simulink model "Simulador"  (R2015a)
settings: Solver=ode45  StartTime=0.0  StopTime=Inf  MaxStep=1  RelTol=1e-3
StopFcn:
  | close all
  | post_simulacion
model workspace (MAT data in the model file):
  m = 3.797
  b = 2.1
  c = 0.3571
  Salar = 0.75
  AR = 5.88
  cg = [0.44 0 0]
  Ix = 1.229
  Iy = 0.1702
  Iz = 0.8808
  Ixz = 0.9343
  e = 0.9935
  alpha0 = 0.267
  coefprop = [0.016415 -0.0142726]
  C_L0 = 0.0254
  C_Lalpha = 4.0191
  C_Lq = 3.8954
  C_Ldelta_e = 0.5872
  C_D0 = 0.0102
  C_Dbeta1 = -2.0864e-07
  C_Dbeta2 = 0.0671
  C_Dq = 0
  C_Ddelta_e = 0.8461
  C_Y0 = 3.2049e-18
  C_Ybeta = -0.1949
  C_Yp = -0.1172
  C_Yr = 0.0959
  C_Ydelta_a = -0.0696
  C_l0 = 1.1518e-18
  C_lbeta = -0.0765
  C_lp = -0.4018
  C_lr = 0.025
  C_ldelta_a = 0.2987
  C_m0 = 0.018
  C_malpha = -0.2524
  C_mq = -1.3047
  C_mdelta_e = -0.4857
  C_n0 = -2.2667e-07
  C_nbeta = 0.0403
  C_np = -0.0247
  C_nr = -0.1252
  C_ndelta_a = 0.0076
  gamma = 0.20958671
  gamma1 = 8.64638926772
  gamma2 = 7.15127867602
  gamma3 = 4.20255654569
  gamma4 = 4.4578208227
  gamma5 = -2.04582843713
  gamma6 = 5.48942420682
  gamma7 = 10.3736620037
  gamma8 = 5.86392142899
  C_p0 = -1.01045424588e-06
  C_pbeta = -0.14184539659
  C_pp = -1.79869539438
  C_pr = -0.45305525336
  C_pdelta_a = 1.28918307845
  C_r0 = -1.3291750703e-06
  C_rbeta = -0.104707259349
  C_rp = -1.93599126586
  C_rr = -0.622717442342
  C_rdelta_a = 1.3761168826
  C_mp = -0.2168
values from neighbouring files (symbols this model uses):
  r = [r_n;r_e;r_d]    [segmento.m]
  waypoints = reshape(waypoints_mat.',[],1)    [plan_de_vuelo.m]
undefined symbols (not defined in the file or in its folder): F, Light, magnitude, MIL, plan_de_vuelo
libraries: simulink_extras x20, aerolibconvert2 x18, aerolibfltsims x2, simulink x2, vrlib x1, instrumentlib x1, aerolibatmos2 x1, aerolibtransform2 x1, aerolibwind2 x1, aerolibgravity2 x1
(part 1 of 3)
settings Model: TunableVars=Velocidad_aerodinamica_AP,Rumbo_AP,Altitud_AP,PalancaTeclado,FMS,GNSS,Viento  TunableVarsStorageClass=Auto,Auto,Auto,Auto,Auto,Auto,Auto  TunableVarsTypeQualifier=,,,,,,  Creator=Cecilia Ruiz Romero  LastModifiedBy=Cecilia Ruiz Romero
settings DataIOCC: TimeSaveName=tiempos

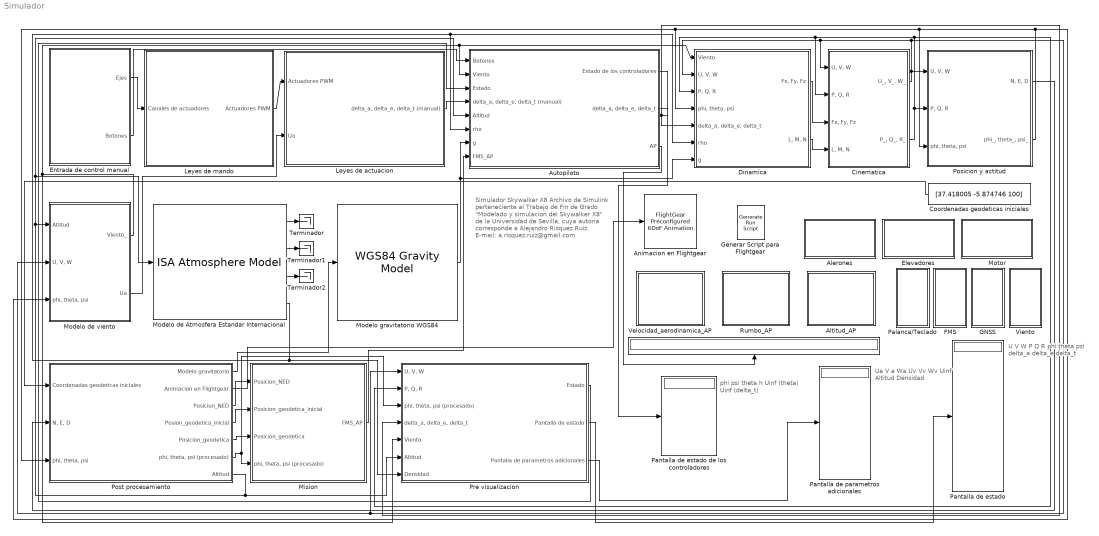
== system Simulador ==
  note: U
      | V
      | W
      | P
      | Q
      | R
      | phi
      | theta
      | psi
      | delta_a
      | delta_e
      | delta_t
  note: Ua
      | V a
      | Wa
      | Uv
      | Vv
      | Wv
      | Uinf
      | Altitud
      | Densidad
  note: phi
      | psi
      | theta
      | h
      | Uinf (theta)
      | Uinf (delta_t)
  note: Simulador Skywalker X8
      |
      | Archivo de Simulink perteneciente al Trabajo de Fin de Grado "Modelado y simulacion del Skywalker X8" de la Universidad de Sevilla, cuya autoria corresponde a Alejandro Risquez Ruiz.
      |
      | E-mail: a.risquez.ruiz@gmail.com
  " " : Display
  Alerones : Subsystem  DialogController=hmiCreateDDGDialog  IsWebBlock=on  mask(MathWorksWebBlock){webBlockId=14687f7d-6eed-453e-adcd-d1944eb0612c, webBlockType=semicirculargauge, ShowInLibBrowser=on, ShowInitialText=on, HMISrcModelName=Simulador}
      mask prompts: webBlockId "WebBlock Id"; webBlockType "WebBlock Type"; HMISrcModelName "Source Model"
      mask Help: helpview([docroot '/mapfiles/simulink.map'], 'hmi_half_gauge')
      mask Display:
      | if strcmp(get_param(bdroot(gcb),'BlockDiagramType'), 'library')
      |     image([(matlabroot) '/toolbox/simulink/hmi/icons/SemicircularGauge.png']);
      | end
  Altitud_AP : Subsystem  DialogController=hmiCreateDDGDialog  IsWebBlock=on  mask(MathWorksWebBlock){webBlockId=223b671f-8fe1-4181-b377-fa138c1070ca, webBlockType=continuousknob, ShowInLibBrowser=on, ShowInitialText=on, HMISrcModelName=Simulador}
      mask prompts: webBlockId "WebBlock Id"; webBlockType "WebBlock Type"; HMISrcModelName "Source Model"
      mask Help: helpview([docroot '/mapfiles/simulink.map'], 'hmi_knob')
      mask Display:
      | if strcmp(get_param(bdroot(gcb),'BlockDiagramType'), 'library')
      |     image([(matlabroot) '/toolbox/simulink/hmi/icons/ContinuousKnob.png']);
      | end
  Animacion en Flightgear : aerolibfltsims/FlightGear Preconfigured 6DoF Animation  xFlightGearVersion=v3.0  DestinationIpAddress=192.168.1.33  DestinationPort=5502  SampleTime=1/30
  Autopiloto : Subsystem
  Cinematica : Subsystem
  Coordenadas geodeticas iniciales : Constant  Value=[37.418005 -5.874746 100]
  Dinamica : Subsystem
  Elevadores : Subsystem  DialogController=hmiCreateDDGDialog  IsWebBlock=on  mask(MathWorksWebBlock){webBlockId=d989d251-72c9-40e1-9d1b-cd89d142c18d, webBlockType=semicirculargauge, ShowInLibBrowser=on, ShowInitialText=on, HMISrcModelName=Simulador}
      mask prompts: webBlockId "WebBlock Id"; webBlockType "WebBlock Type"; HMISrcModelName "Source Model"
      mask Help: helpview([docroot '/mapfiles/simulink.map'], 'hmi_half_gauge')
      mask Display:
      | if strcmp(get_param(bdroot(gcb),'BlockDiagramType'), 'library')
      |     image([(matlabroot) '/toolbox/simulink/hmi/icons/SemicircularGauge.png']);
      | end
  Entrada de control manual : Subsystem
  FMS : Subsystem  DialogController=hmiCreateDDGDialog  IsWebBlock=on  mask(MathWorksWebBlock){webBlockId=f65861c9-849a-4d55-a765-84128246603e, webBlockType=toggleswitch, ShowInLibBrowser=on, ShowInitialText=on, HMISrcModelName=Simulador}
      mask prompts: webBlockId "WebBlock Id"; webBlockType "WebBlock Type"; HMISrcModelName "Source Model"
      mask Help: helpview([docroot '/mapfiles/simulink.map'], 'hmi_toggle_switch')
      mask Display:
      | if strcmp(get_param(bdroot(gcb),'BlockDiagramType'), 'library')
      |     image([(matlabroot) '/toolbox/simulink/hmi/icons/ToggleSwitch.png']);
      | end
  GNSS : Subsystem  DialogController=hmiCreateDDGDialog  IsWebBlock=on  mask(MathWorksWebBlock){webBlockId=2f82c36a-ef1f-4a61-96ee-8f2028b7861b, webBlockType=toggleswitch, ShowInLibBrowser=on, ShowInitialText=on, HMISrcModelName=Simulador}
      mask prompts: webBlockId "WebBlock Id"; webBlockType "WebBlock Type"; HMISrcModelName "Source Model"
      mask Help: helpview([docroot '/mapfiles/simulink.map'], 'hmi_toggle_switch')
      mask Display:
      | if strcmp(get_param(bdroot(gcb),'BlockDiagramType'), 'library')
      |     image([(matlabroot) '/toolbox/simulink/hmi/icons/ToggleSwitch.png']);
      | end
  Generar Script para Flightgear : aerolibfltsims/Generate Run Script  OutputFileName=Flightgear_simulador.bat  FlightGearBaseDirectory=C:\Program Files\FlightGear  GeometryModelName=Malolo1  DestinationPort=5502  OriginAddress=192.168.1.34  OriginPort=5505  LocalAddress=192.168.1.35  AirportId=LEZL  RunwayId=27  InitialAltitude=328  InitialHeading=270  OffsetDistance=0  OffsetAzimuth=0  GenerateFile=off  Architecture=Win64  dataFlow=Receive
  Leyes de actuacion : Subsystem
  Leyes de mando : Subsystem
  Mision : Subsystem
  Modelo de Atmosfera Estandar Internacional : aerolibatmos2/ISA Atmosphere Model  custom=off  g=9.80665  gamma=1.4  R=287.0531  L=0.0065  h_trop=11000  h_strat=20000  rho0=1.225  P0=101325  T0=288.15  h0=0
  Modelo de viento : Subsystem
  Modelo gravitatorio WGS84 : aerolibgravity2/WGS84 Gravity Model   model=WGS84 Taylor Series  units=Metric (MKS)  no_atmos=on  precessing=on  jd_loc=off  month=October  day=10  year=2004  no_centrifugal=on  action=Warning
  Motor : Subsystem  DialogController=hmiCreateDDGDialog  IsWebBlock=on  mask(MathWorksWebBlock){webBlockId=dc943369-9c23-4275-9e07-e512671338e7, webBlockType=semicirculargauge, ShowInLibBrowser=on, ShowInitialText=on, HMISrcModelName=Simulador}
      mask prompts: webBlockId "WebBlock Id"; webBlockType "WebBlock Type"; HMISrcModelName "Source Model"
      mask Help: helpview([docroot '/mapfiles/simulink.map'], 'hmi_half_gauge')
      mask Display:
      | if strcmp(get_param(bdroot(gcb),'BlockDiagramType'), 'library')
      |     image([(matlabroot) '/toolbox/simulink/hmi/icons/SemicircularGauge.png']);
      | end
  Palanca/Teclado : Subsystem  DialogController=hmiCreateDDGDialog  IsWebBlock=on  mask(MathWorksWebBlock){webBlockId=b63e11f2-ce41-4b45-96ee-a8e10d270359, webBlockType=toggleswitch, ShowInLibBrowser=on, ShowInitialText=on, HMISrcModelName=Simulador}
      mask prompts: webBlockId "WebBlock Id"; webBlockType "WebBlock Type"; HMISrcModelName "Source Model"
      mask Help: helpview([docroot '/mapfiles/simulink.map'], 'hmi_toggle_switch')
      mask Display:
      | if strcmp(get_param(bdroot(gcb),'BlockDiagramType'), 'library')
      |     image([(matlabroot) '/toolbox/simulink/hmi/icons/ToggleSwitch.png']);
      | end
  Pantalla de estado : Display
  Pantalla de estado de los controladores : Display
  Pantalla de parametros adicionales : Display
  Posicion y actitud : Subsystem
  Post procesamiento : Subsystem
  Pre visualizacion : Subsystem
  Rumbo_AP : Subsystem  DialogController=hmiCreateDDGDialog  IsWebBlock=on  mask(MathWorksWebBlock){webBlockId=9d5373b8-7b64-41e6-bd7e-2392d6322634, webBlockType=continuousknob, ShowInLibBrowser=on, ShowInitialText=on, HMISrcModelName=Simulador}
      mask prompts: webBlockId "WebBlock Id"; webBlockType "WebBlock Type"; HMISrcModelName "Source Model"
      mask Help: helpview([docroot '/mapfiles/simulink.map'], 'hmi_knob')
      mask Display:
      | if strcmp(get_param(bdroot(gcb),'BlockDiagramType'), 'library')
      |     image([(matlabroot) '/toolbox/simulink/hmi/icons/ContinuousKnob.png']);
      | end
  Terminador : Terminator
  Terminador1 : Terminator
  Terminador2 : Terminator
  Velocidad_aerodinamica_AP : Subsystem  DialogController=hmiCreateDDGDialog  IsWebBlock=on  mask(MathWorksWebBlock){webBlockId=5a147658-4b96-4464-a5e7-82583d5f87ac, webBlockType=continuousknob, ShowInLibBrowser=on, ShowInitialText=on, HMISrcModelName=Simulador}
      mask prompts: webBlockId "WebBlock Id"; webBlockType "WebBlock Type"; HMISrcModelName "Source Model"
      mask Help: helpview([docroot '/mapfiles/simulink.map'], 'hmi_knob')
      mask Display:
      | if strcmp(get_param(bdroot(gcb),'BlockDiagramType'), 'library')
      |     image([(matlabroot) '/toolbox/simulink/hmi/icons/ContinuousKnob.png']);
      | end
  Viento : Subsystem  DialogController=hmiCreateDDGDialog  IsWebBlock=on  mask(MathWorksWebBlock){webBlockId=de649073-e8b6-4552-a188-ccf5b7e05afd, webBlockType=toggleswitch, ShowInLibBrowser=on, ShowInitialText=on, HMISrcModelName=Simulador}
      mask prompts: webBlockId "WebBlock Id"; webBlockType "WebBlock Type"; HMISrcModelName "Source Model"
      mask Help: helpview([docroot '/mapfiles/simulink.map'], 'hmi_toggle_switch')
      mask Display:
      | if strcmp(get_param(bdroot(gcb),'BlockDiagramType'), 'library')
      |     image([(matlabroot) '/toolbox/simulink/hmi/icons/ToggleSwitch.png']);
      | end
  wires:
  Entrada de control manual/1(Ejes) -> Leyes de mando/1(Canales de actuadores)
  Entrada de control manual/2(Botones) -> Autopiloto/1(Botones)
  Leyes de mando/1(Actuadores PWM) -> Leyes de actuacion/1(Actuadores PWM)
  Modelo de Atmosfera Estandar Internacional/1 -> Terminador/1
  Modelo de Atmosfera Estandar Internacional/2 -> Terminador1/1
  Modelo de Atmosfera Estandar Internacional/3 -> Terminador2/1
  Pre visualizacion/1(Estado) -> Autopiloto/3(Estado)
  Leyes de actuacion/1("delta_a, delta_e, delta_t (manual)") -> Autopiloto/4("delta_a, delta_e, delta_t (manual)")
  Post procesamiento/7(Altitud) -> Modelo de viento/1(Altitud), Modelo de Atmosfera Estandar Internacional/1, Autopiloto/5(Altitud), Pre visualizacion/6(Altitud)
  Mision/1(FMS_AP) -> Autopiloto/8(FMS_AP)
  Autopiloto/2("delta_a, delta_e, delta_t") -> Pre visualizacion/4("delta_a, delta_e, delta_t"), Dinamica/5("delta_a, delta_e, delta_t")
  Cinematica/1("U_, V_, W_") -> Posicion y actitud/1("U, V, W"), Modelo de viento/2("U, V, W"), Pre visualizacion/1("U, V, W"), Cinematica/1("U, V, W"), Dinamica/2("U, V, W")
  Modelo de viento/1(Viento_) -> Pre visualizacion/5(Viento), Dinamica/1(Viento), Autopiloto/2(Viento)
  Modelo de Atmosfera Estandar Internacional/4 -> Pre visualizacion/7(Densidad), Dinamica/6(rho), Autopiloto/6(rho)
  Autopiloto/1(Estado de los controladores) -> Pantalla de estado de los controladores/1
  Cinematica/2("P_, Q_, R_") -> Posicion y actitud/2("P, Q, R"), Pre visualizacion/2("P, Q, R"), Cinematica/2("P, Q, R"), Dinamica/3("P, Q, R")
  Posicion y actitud/2("phi_, theta_, psi_") -> Posicion y actitud/3("phi, theta, psi"), Dinamica/4("phi, theta, psi"), Post procesamiento/3("phi, theta, psi"), Modelo de viento/3("phi, theta, psi")
  Autopiloto/3(AP) -> " "/1
  Dinamica/1("Fx, Fy, Fz") -> Cinematica/3("Fx, Fy, Fz")
  Dinamica/2("L, M, N") -> Cinematica/4("L, M, N")
  Posicion y actitud/1("N, E, D") -> Post procesamiento/2("N, E, D")
  Coordenadas geodeticas iniciales/1 -> Post procesamiento/1(Coordenadas geodeticas iniciales)
  Post procesamiento/2(Animacion en Flightgear) -> Animacion en Flightgear/1
  Post procesamiento/3(Posicion_NED) -> Mision/1(Posicion_NED)
  Post procesamiento/4(Posion_geodetica_inicial) -> Mision/2(Posicion_geodetica_inicial)
  Post procesamiento/5(Posicion_geodetica) -> Mision/3(Posicion_geodetica)
  Post procesamiento/6("phi, theta, psi (procesado)") -> Mision/4("phi, theta, psi (procesado)"), Pre visualizacion/3("phi, theta, psi (procesado)")
  Pre visualizacion/2(Pantalla de estado) -> Pantalla de estado/1
  Pre visualizacion/3(Pantalla de parametros adicionales) -> Pantalla de parametros adicionales/1
  Modelo de viento/2(Ua) -> Leyes de actuacion/2(Ua)
  Modelo gravitatorio WGS84/1 -> Dinamica/7(g), Autopiloto/7(g)
  Post procesamiento/1(Modelo gravitatorio) -> Modelo gravitatorio WGS84/1

== system Simulador/Alerones ==

== system Simulador/Altitud_AP ==

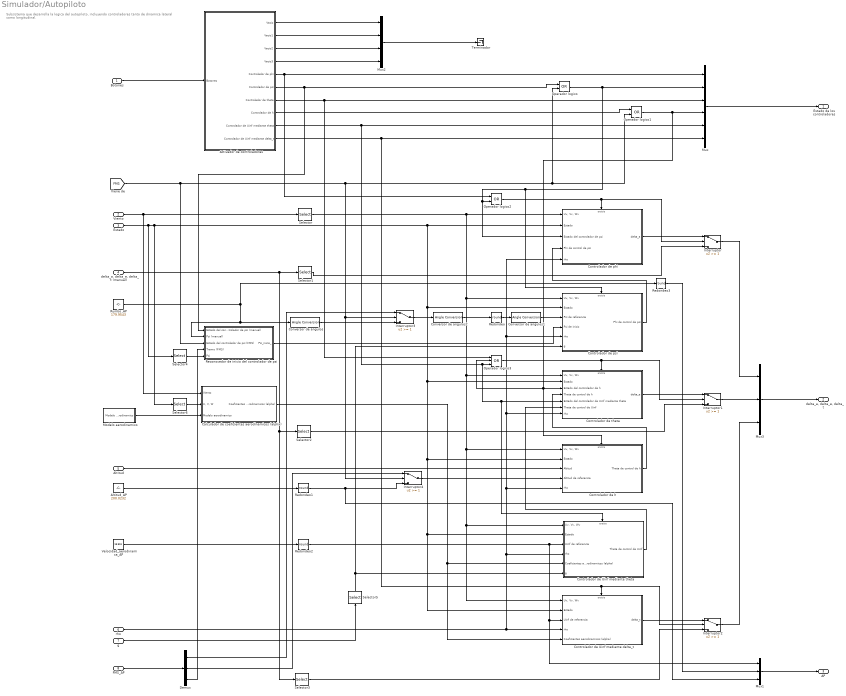
== system Simulador/Autopiloto ==
  note: Subsistema que desarrolla la logica del
      | autopiloto, incluyendo controladores tanto
      | de dinamica lateral como longitudinal.
  Botones : Inport
  Viento : Inport  Port=2
  Estado : Inport  Port=3
  "delta_a, delta_e, delta_t (manual)" : Inport  Port=4
  Altitud : Inport  Port=5
  rho : Inport  Port=6
  g : Inport  Port=7
  FMS_AP : Inport  Port=8
  Activador de controladores : Subsystem
  Altitud_AP : Constant  Value=200.0232
  Calculador de coeficientes aerodinamicos (alpha) : Subsystem
  Controlador de Uinf mediante delta_t : Subsystem
  Controlador de Uinf mediante theta : Subsystem
  Controlador de h : Subsystem
  Controlador de phi : Subsystem
  Controlador de psi : Subsystem
  Controlador de theta : Subsystem
  Conversor de angulos : aerolibconvert2/Angle Conversion  IU=deg  OU=rad
  Conversor de angulos1 : aerolibconvert2/Angle Conversion  IU=deg  OU=rad
  Conversor de angulos2 : aerolibconvert2/Angle Conversion  IU=rad  OU=deg
  Demux : Demux  Outputs=3
  Interruptor{,1..4} (5 alike) : Switch  Threshold=1
  Modelo aerodinamico : Subsystem
  Mux : Mux  Inputs=6
  Mux1 : Mux  Inputs=3
  Mux2 : Mux
  Mux3 : Mux  Inputs=3
  Operador logico : Logic  Operator=OR  AllPortsSameDT=off  OutDataTypeStr=boolean
  Operador logico1 : Logic  Operator=OR  AllPortsSameDT=off  OutDataTypeStr=boolean
  Operador logico2 : Logic  Operator=OR  AllPortsSameDT=off  OutDataTypeStr=boolean
  Operador logico3 : Logic  Operator=OR  Inputs=3  AllPortsSameDT=off  OutDataTypeStr=boolean
  Reconocedor de inicio del controlador de psi : Subsystem
  Redondeo{,1..3} (4 alike) : Rounding  Operator=round
  Rumbo_AP : Constant  Value=179.9543
  Selector : Selector  InputPortWidth=6  Indices=[1 2 3]
  Selector1 : Selector  InputPortWidth=3
  Selector2 : Selector  InputPortWidth=3  Indices=2
  Selector3 : Selector  InputPortWidth=3  Indices=3
  Selector4 : Selector  InputPortWidth=12  Indices=9
  Selector5 : Selector  InputPortWidth=3  Indices=3
  Selector6 : Selector  InputPortWidth=12  Indices=[1 2 3]
  Terminador : Terminator
  Velocidad_aerodinamica_AP : Constant  Value=19.919
  Estado de los controladores : Outport
  "delta_a, delta_e, delta_t" : Outport  Port=2
  AP : Outport  Port=3
  wires:
  Botones/1 -> Activador de controladores/1(Botones)
  Mux1/1 -> AP/1
  Altitud_AP/1 -> Redondeo1/1
  [FMS] -> Operador logico1/2, Operador logico/2, Interruptor4/2, Interruptor3/2, Reconocedor de inicio del controlador de psi/3(Estado del controlador de psi (FMS))
  Activador de controladores/9(Controlador de Uinf mediante theta) -> Mux/5, Controlador de theta/5(Estado del controlador de Uinf mediante theta), Controlador de Uinf mediante theta/Enable, Operador logico3/3
  Activador de controladores/8(Controlador de h) -> Operador logico1/1
  Activador de controladores/7(Controlador de theta) -> Mux/3, Operador logico3/1
  Activador de controladores/5(Controlador de phi) -> Mux/1, Operador logico2/1
  Activador de controladores/6(Controlador de psi) -> Operador logico/1, Reconocedor de inicio del controlador de psi/1(Estado del controlador de psi (manual))
  Activador de controladores/1(Vacio) -> Mux2/1
  Activador de controladores/2(Vacio1) -> Mux2/2
  Activador de controladores/3(Vacio2) -> Mux2/3
  Activador de controladores/4(Vacio3) -> Mux2/4
  Mux2/1 -> Terminador/1
  Mux/1 -> Estado de los controladores/1
  Viento/1 -> Calculador de coeficientes aerodinamicos (alpha)/1(Viento), Selector/1
  Estado/1 -> Selector6/1, Controlador de Uinf mediante delta_t/2("Estado "), Controlador de Uinf mediante theta/2("Estado "), Controlador de h/2("Estado "), Controlador de theta/2("Estado "), Controlador de psi/2("Estado "), Controlador de phi/2("Estado "), Selector4/1
  Selector/1 -> Controlador de Uinf mediante delta_t/1("Uv, Vv, Wv"), Controlador de Uinf mediante theta/1("Uv, Vv, Wv"), Controlador de h/1("Uv, Vv, Wv"), Controlador de theta/1("Uv, Vv, Wv"), Controlador de psi/1("Uv, Vv, Wv"), Controlador de phi/1("Uv, Vv, Wv")
  Operador logico2/1 -> Interruptor/2, Controlador de phi/Enable
  Controlador de phi/1(delta_a) -> Interruptor/1
  "delta_a, delta_e, delta_t (manual)"/1 -> Selector1/1, Selector2/1, Selector3/1
  Selector1/1 -> Interruptor/3
  Controlador de psi/1(Phi de control de psi) -> Controlador de phi/4(Phi de control de psi)
  Operador logico3/1 -> Interruptor1/2, Controlador de theta/Enable
  Controlador de theta/1(delta_e) -> Interruptor1/1
  Selector2/1 -> Interruptor1/3
  rho/1 -> Controlador de Uinf mediante delta_t/4(rho), Controlador de h/5(rho), Controlador de theta/7(rho), Controlador de psi/5(rho), Controlador de phi/5(rho), Controlador de Uinf mediante theta/4(rho)
  Controlador de h/1(Theta de control de h) -> Controlador de theta/4(Theta de control de h)
  Redondeo2/1 -> Mux1/1, Controlador de Uinf mediante delta_t/3(Uinf de referencia), Controlador de Uinf mediante theta/3(Uinf de referencia)
  Velocidad_aerodinamica_AP/1 -> Redondeo2/1
  Activador de controladores/10(Controlador de Uinf mediante delta_t) -> Mux/6, Controlador de Uinf mediante delta_t/Enable, Interruptor2/2
  Controlador de Uinf mediante delta_t/1(delta_t) -> Interruptor2/1
  Selector3/1 -> Interruptor2/3
  Controlador de Uinf mediante theta/1(Theta de control de Uinf) -> Controlador de theta/6(Theta de control de Uinf)
  Altitud/1 -> Controlador de h/3(Altitud)
  Interruptor4/1 -> Controlador de h/4(Altitud de referencia)
  Mux3/1 -> "delta_a, delta_e, delta_t"/1
  Interruptor2/1 -> Mux3/3
  Interruptor1/1 -> Mux3/2
  Interruptor/1 -> Mux3/1
  Redondeo1/1 -> Mux1/3, Interruptor4/3
  Redondeo3/1 -> Mux1/2
  FMS_AP/1 -> Demux/1
  Rumbo_AP/1 -> Redondeo3/1, Conversor de angulos/1, Reconocedor de inicio del controlador de psi/2(Psi (manual))
  Selector4/1 -> Reconocedor de inicio del controlador de psi/5(Psi)
  Reconocedor de inicio del controlador de psi/1(Psi_inicio_) -> Controlador de psi/4(Psi de inicio)
  Operador logico/1 -> Mux/2, Operador logico2/2, Controlador de phi/3(Estado del controlador de psi), Controlador de psi/Enable
  Operador logico1/1 -> Controlador de theta/3(Estado del controlador de h), Operador logico3/2, Controlador de h/Enable, Mux/4
  Conversor de angulos1/1 -> Controlador de psi/3(Psi de referencia)
  Redondeo/1 -> Conversor de angulos1/1
  Conversor de angulos/1 -> Interruptor3/3
  Conversor de angulos2/1 -> Redondeo/1
  Interruptor3/1 -> Conversor de angulos2/1
  g/1 -> Selector5/1
  Selector5/1 -> Controlador de psi/6(g), Controlador de Uinf mediante theta/6(g)
  Modelo aerodinamico/1(Modelo aerodinamico) -> Calculador de coeficientes aerodinamicos (alpha)/3(Modelo aerodinamico)
  Selector6/1 -> Calculador de coeficientes aerodinamicos (alpha)/2("U, V, W")
  Calculador de coeficientes aerodinamicos (alpha)/1(Coeficientes aerodinamicos (alpha)) -> Controlador de Uinf mediante delta_t/5(Coeficientes aerodinamicos (alpha)), Controlador de Uinf mediante theta/5(Coeficientes aerodinamicos (alpha))
  Demux/3 -> Reconocedor de inicio del controlador de psi/4(Tramo (FMS))
  Demux/1 -> Interruptor3/1
  Demux/2 -> Interruptor4/1

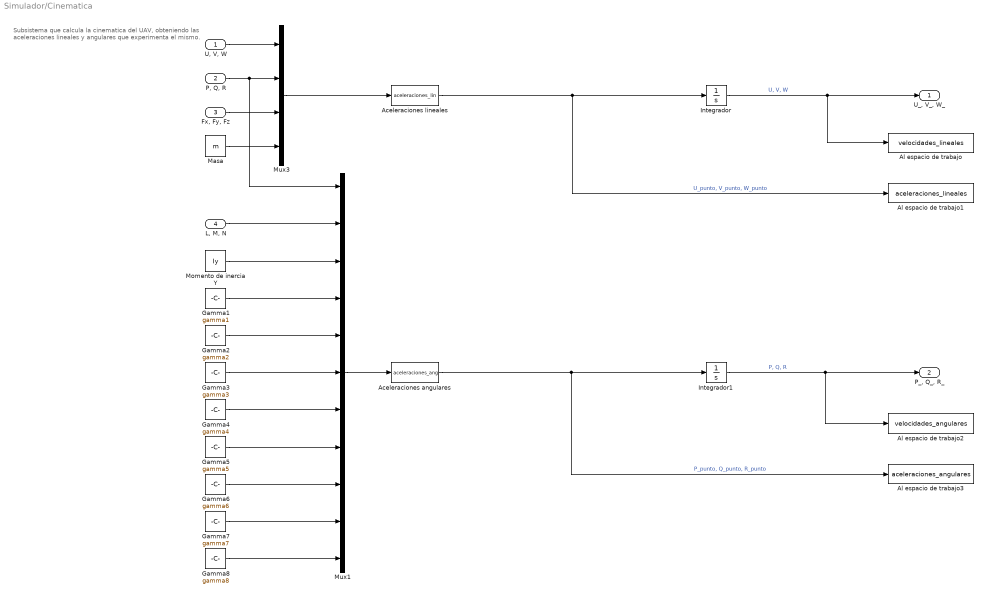
== system Simulador/Cinematica ==
  note: Subsistema que calcula la cinematica del
      | UAV, obteniendo las aceleraciones lineales
      | y angulares que experimenta el mismo.
  "U, V, W" : Inport
  "P, Q, R" : Inport  Port=2
  "Fx, Fy, Fz" : Inport  Port=3
  "L, M, N" : Inport  Port=4
  Aceleraciones angulares : MATLABFcn  MATLABFcn=aceleraciones_ang  OutputDimensions=3
  Aceleraciones lineales : MATLABFcn  MATLABFcn=aceleraciones_lin  OutputDimensions=3
  Al espacio de trabajo : ToWorkspace  VariableName=velocidades_lineales  SaveFormat=Timeseries  SampleTime=-1
  Al espacio de trabajo1 : ToWorkspace  VariableName=aceleraciones_lineales  SaveFormat=Timeseries  SampleTime=-1
  Al espacio de trabajo2 : ToWorkspace  VariableName=velocidades_angulares  SaveFormat=Timeseries  SampleTime=-1
  Al espacio de trabajo3 : ToWorkspace  VariableName=aceleraciones_angulares  SaveFormat=Timeseries  SampleTime=-1
  Gamma1 : Constant  Value=gamma1
  Gamma2 : Constant  Value=gamma2
  Gamma3 : Constant  Value=gamma3
  Gamma4 : Constant  Value=gamma4
  Gamma5 : Constant  Value=gamma5
  Gamma6 : Constant  Value=gamma6
  Gamma7 : Constant  Value=gamma7
  Gamma8 : Constant  Value=gamma8
  Integrador : Integrator  InitialCondition=[22.5000 1.20777e-04 0.678706]
  Integrador1 : Integrator  InitialCondition=[-6.87125e-22 -3.91163e-24 -2.13625e-23]
  Masa : Constant  Value=m
  Momento de inercia Y : Constant  Value=Iy
  Mux1 : Mux  Inputs=11
  Mux3 : Mux
  "U_, V_, W_" : Outport
  "P_, Q_, R_" : Outport  Port=2
  wires:
  Aceleraciones lineales/1 -> Integrador/1, Al espacio de trabajo1/1  "U_punto, V_punto, W_punto"
  Aceleraciones angulares/1 -> Integrador1/1, Al espacio de trabajo3/1  "P_punto, Q_punto, R_punto"
  "U, V, W"/1 -> Mux3/1
  "P, Q, R"/1 -> Mux3/2, Mux1/1
  "Fx, Fy, Fz"/1 -> Mux3/3
  "L, M, N"/1 -> Mux1/2
  Mux3/1 -> Aceleraciones lineales/1
  Mux1/1 -> Aceleraciones angulares/1
  Integrador/1 -> "U_, V_, W_"/1, Al espacio de trabajo/1  "U, V, W"
  Integrador1/1 -> "P_, Q_, R_"/1, Al espacio de trabajo2/1  "P, Q, R"
  Momento de inercia Y/1 -> Mux1/3
  Gamma1/1 -> Mux1/4
  Gamma2/1 -> Mux1/5
  Gamma3/1 -> Mux1/6
  Gamma4/1 -> Mux1/7
  Gamma5/1 -> Mux1/8
  Gamma6/1 -> Mux1/9
  Gamma7/1 -> Mux1/10
  Gamma8/1 -> Mux1/11
  Masa/1 -> Mux3/4

== system Simulador/Dinamica ==
  note: Subsistema que calcula la dinamica
      | del UAV, obteniendo las fuerzas y
      | momentos ejercidos sobre el mismo.
  Viento : Inport
  "U, V, W" : Inport  Port=2
  "P, Q, R" : Inport  Port=3
  "phi, theta, psi" : Inport  Port=4
  "delta_a, delta_e, delta_t" : Inport  Port=5
  rho : Inport  Port=6
  g : Inport  Port=7
  Al espacio de trabajo : ToWorkspace  VariableName=fuerzas  SaveFormat=Timeseries  SampleTime=-1
  Al espacio de trabajo1 : ToWorkspace  VariableName=momentos  SaveFormat=Timeseries  SampleTime=-1
  Calculador de coeficientes aerodinamicos : Subsystem
  Fuerzas : MATLABFcn  MATLABFcn=fuerzas  OutputDimensions=3
  Modelo aerodinamico : Subsystem
  Momentos : MATLABFcn  MATLABFcn=momentos  OutputDimensions=3
  Mux1 : Mux  Inputs=10
  Mux5 : Mux  Inputs=6
  Selector : Selector  InputPortWidth=6  Indices=[1 2 3]
  Selector1 : Selector  InputPortWidth=3  Indices=3
  Selector2 : Selector  InputPortWidth=3  Indices=3
  Selector3 : Selector  InputPortWidth=35
  Selector4 : Selector  InputPortWidth=35  Indices=4
  Selector5 : Selector  InputPortWidth=6  Indices=[4 5 6]
  Selector6 : Selector  InputPortWidth=35  Indices=2
  Selector7 : Selector  InputPortWidth=35  Indices=3
  "Fx, Fy, Fz" : Outport
  "L, M, N" : Outport  Port=2
  wires:
  Fuerzas/1 -> "Fx, Fy, Fz"/1, Al espacio de trabajo/1  "Fx, Fy, Fz"
  Momentos/1 -> "L, M, N"/1, Al espacio de trabajo1/1  "L, M, N"
  g/1 -> Selector2/1
  "delta_a, delta_e, delta_t"/1 -> Selector1/1, Calculador de coeficientes aerodinamicos/4("delta_a, delta_e, delta_t")
  Viento/1 -> Calculador de coeficientes aerodinamicos/1(Viento)
  "U, V, W"/1 -> Calculador de coeficientes aerodinamicos/2("U, V, W")
  "P, Q, R"/1 -> Calculador de coeficientes aerodinamicos/3("P, Q, R")
  Calculador de coeficientes aerodinamicos/4(Coeficientes aerodinamicos) -> Selector/1, Selector5/1
  rho/1 -> Mux5/3, Mux1/7
  Mux1/1 -> Fuerzas/1
  Mux5/1 -> Momentos/1
  Modelo aerodinamico/1(Modelo aerodinamico) -> Selector7/1, Selector6/1, Selector4/1, Selector3/1, Calculador de coeficientes aerodinamicos/5(Modelo aerodinamico)
  Selector4/1 -> Mux5/6, Mux1/10
  Calculador de coeficientes aerodinamicos/1(alpha) -> Mux1/1
  Calculador de coeficientes aerodinamicos/2(beta) -> Mux1/2
  Selector/1 -> Mux1/4
  Calculador de coeficientes aerodinamicos/3(Uinf) -> Mux5/1, Mux1/3
  "phi, theta, psi"/1 -> Mux1/5
  Selector1/1 -> Mux1/6
  Selector2/1 -> Mux1/8
  Selector3/1 -> Mux1/9
  Selector7/1 -> Mux5/5
  Selector6/1 -> Mux5/4
  Selector5/1 -> Mux5/2

== system Simulador/Elevadores ==

== system Simulador/Entrada de control manual ==
  note: Subsistema que toma como entrada de control manual del UAV la palanca de mando o el teclado en funcion de la
      | posicion del interruptor Palanca/Teclado .
  Constante : Constant  Value=50
  Constante1 : Constant
  Constante2 : Constant  Value=-50
  Constante3 : Constant  Value=[0 0 0]
  Demux : Demux  Outputs=3
  Interruptor : Switch  Criteria=u2 ~= 0
  Interruptor1 : Switch  Criteria=u2 ~= 0
  Operador logico : Logic  Operator=NOT  AllPortsSameDT=off  OutDataTypeStr=boolean
  Operador logico1 : Logic  Operator=OR  AllPortsSameDT=off  OutDataTypeStr=boolean
  Palanca de mando : Subsystem  TreatAsAtomicUnit=on
  PalancaTeclado : Constant  OutDataTypeStr=boolean
  Producto : Product
  Producto1 : Product
  Producto2 : Product
  Sum : Sum  Inputs=|++
  Sum1 : Sum  Inputs=|+-
  Teclado : Subsystem  TreatAsAtomicUnit=on
  Terminador : Terminator
  Terminador1 : Terminator
  Terminador2 : Terminator
  Ejes : Outport
  Botones : Outport  Port=2
  tag scope: Entrada=global
  wires:
  PalancaTeclado/1 -> Operador logico/1, Palanca de mando/Enable, Interruptor1/2, Interruptor/2, [Entrada]
  Operador logico/1 -> Teclado/Enable
  Sum/1 -> Demux/1, Ejes/1
  Palanca de mando/2(Botones) -> Operador logico1/1
  Teclado/2(Botones) -> Operador logico1/2
  Operador logico1/1 -> Botones/1
  Demux/3 -> Sum1/1
  Constante1/1 -> Sum1/2
  Sum1/1 -> Producto2/1
  Constante2/1 -> Producto2/2
  Producto2/1 -> Terminador2/1
  Demux/1 -> Producto/1
  Demux/2 -> Producto1/1
  Constante/1 -> Producto1/2, Producto/2
  Producto1/1 -> Terminador1/1
  Producto/1 -> Terminador/1
  Interruptor/1 -> Sum/1
  Palanca de mando/1(Ejes) -> Interruptor/1
  Teclado/1(Ejes) -> Interruptor1/3
  Constante3/1 -> Interruptor/3, Interruptor1/1
  Interruptor1/1 -> Sum/2

== system Simulador/FMS ==

== system Simulador/GNSS ==

== system Simulador/Leyes de actuacion ==
  note: Subsistema que define las leyes de actuacion
      | del UAV, permitiendo obtener los grados de
      | deflexion de las diferentes superficies de control
      | asi como la fuerza que ejerce la planta motor.
  Actuadores PWM : Inport
  Ua : Inport  Port=2
  Al espacio de trabajo : ToWorkspace  VariableName=deflexion_alerones  SaveFormat=Timeseries  SampleTime=-1
  Al espacio de trabajo1 : ToWorkspace  VariableName=deflexion_elevadores  SaveFormat=Timeseries  SampleTime=-1
  Al espacio de trabajo2 : ToWorkspace  VariableName=fuerza_motor  SaveFormat=Timeseries  SampleTime=-1
  Conversor de angulos : aerolibconvert2/Angle Conversion  IU=rad  OU=deg
  Conversor de angulos1 : aerolibconvert2/Angle Conversion  IU=rad  OU=deg
  Demux : Demux  Outputs=3
  Ley de alerones : Subsystem
  Ley de elevadores : Subsystem
  Ley de propulsion : Subsystem
  Mux : Mux  Inputs=3
  "delta_a, delta_e, delta_t (manual)" : Outport
  wires:
  Ley de propulsion/1(delta_t) -> Al espacio de trabajo2/1, Mux/3
  Ua/1 -> Ley de propulsion/2(Ua)
  Ley de alerones/1(delta_a) -> Conversor de angulos/1, Mux/1
  Ley de elevadores/1(delta_e) -> Conversor de angulos1/1, Mux/2
  Conversor de angulos/1 -> Al espacio de trabajo/1
  Conversor de angulos1/1 -> Al espacio de trabajo1/1
  Demux/2 -> Ley de elevadores/1(Elevadores PWM)
  Demux/3 -> Ley de propulsion/1(Motor PWM)
  Demux/1 -> Ley de alerones/1(Alerones PWM)
  Actuadores PWM/1 -> Demux/1
  Mux/1 -> "delta_a, delta_e, delta_t (manual)"/1

== system Simulador/Leyes de mando ==
  note: Subsistema que convierte la señal lineal de entrada manual proveniente del joystick o del teclado en una cubica de tal manera que recrea una zona muerta entorno al punto de calibracion.
  Canales de actuadores : Inport
  Constante : Constant  Value=1520
  Constante1 : Constant  Value=1520
  Constante3 : Constant  Value=1600
  Demux : Demux  Outputs=3
  Ganancia : Gain  Gain=580
  Ganancia1 : Gain  Gain=580
  Ganancia2 : Gain  Gain=-500
  Mux : Mux  Inputs=3
  Producto : Product  Inputs=3
  Producto1 : Product  Inputs=3
  Sum : Sum  Inputs=|++
  Sum1 : Sum  Inputs=|++
  Sum2 : Sum  Inputs=|++
  Actuadores PWM : Outport
  wires:
  Ganancia2/1 -> Sum/1
  Constante3/1 -> Sum/2
  Ganancia/1 -> Sum1/1
  Constante/1 -> Sum1/2
  Ganancia1/1 -> Sum2/1
  Constante1/1 -> Sum2/2
  Producto/1 -> Ganancia/1
  Producto1/1 -> Ganancia1/1
  Demux/2 -> Producto1/3, Producto1/2, Producto1/1  "Canal elevadores"
  Canales de actuadores/1 -> Demux/1
  Demux/3 -> Ganancia2/1  "Canal motor"
  Demux/1 -> Producto/1, Producto/2, Producto/3  "Canal alerones"
  Sum2/1 -> Mux/2  "Elevadores PWM"
  Sum/1 -> Mux/3  "Motor PWM"
  Sum1/1 -> Mux/1  "Alerones PWM"
  Mux/1 -> Actuadores PWM/1

== system Simulador/Mision ==
  note: Subsistema que desarrolla la logica del bloque
      | de mision, incluyendo un sistema de gestion
      | del vuelo asi como un receptor de un
      | sistema de posicionamiento por satelite.
  Posicion_NED : Inport
  Posicion_geodetica_inicial : Inport  Port=2
  Posicion_geodetica : Inport  Port=3  SampleTime=1
  "phi, theta, psi (procesado)" : Inport  Port=4  SampleTime=1
  Al espacio de trabajo : ToWorkspace  VariableName=posicion_geodetica  SaveFormat=Timeseries  SampleTime=-1
  Conversor de angulos : aerolibconvert2/Angle Conversion  IU=rad  OU=deg
  FMS : Constant  Value=0  OutDataTypeStr=double
  GNSS : Constant  Value=0
  Gestor de GPS : Subsystem
  Gestor de trayectorias : Subsystem  InitFcn=plan_de_vuelo;
  Reconocedor de reinicio de FMS : Subsystem
  Selector : Selector  InputPortWidth=3  Indices=3
  FMS_AP : Outport
  tag scope: FMS=global
  wires:
  "phi, theta, psi (procesado)"/1 -> Conversor de angulos/1
  Gestor de trayectorias/1(FMS_AP) -> FMS_AP/1
  FMS/1 -> [FMS], Gestor de trayectorias/Enable, Reconocedor de reinicio de FMS/1(FMS)
  GNSS/1 -> Gestor de GPS/Enable
  Posicion_geodetica_inicial/1 -> Gestor de trayectorias/2(Posicion_geodetica_inicial)
  Reconocedor de reinicio de FMS/2(Posicion_NED_reinicio) -> Gestor de trayectorias/4(Posicion_NED_reinicio)
  Posicion_NED/1 -> Reconocedor de reinicio de FMS/2(Posicion_NED), Gestor de trayectorias/1(Posicion_NED)
  Reconocedor de reinicio de FMS/1(Disparo) -> Gestor de trayectorias/5(Reinicio_disparador)
  Conversor de angulos/1 -> Selector/1
  Selector/1 -> Gestor de trayectorias/3(Psi), Gestor de GPS/2("Psi ")
  Posicion_geodetica/1 -> Al espacio de trabajo/1, Gestor de GPS/1(Posicion_geodetica)

== system Simulador/Modelo de viento ==
  note: Subsistema que implementa el
      | modelo de viento en el simulador.
  Altitud : Inport
  "U, V, W" : Inport  Port=2
  "phi, theta, psi" : Inport  Port=3
  Constante : Constant
  Constante1 : Constant  Value=0
  Interruptor : Switch  Criteria=u2 ~= 0
  Modulo de V_total : Subsystem
  Mux : Mux  Inputs=2
  Producto : Product
  R_nb : aerolibtransform2/Rotation Angles to Direction Cosine Matrix  rotationOrder=ZYX
  Selector : Selector  InputPortWidth=3
  Subsistema de modelo de viento : Subsystem  TreatAsAtomicUnit=on
  Sum : Sum  Inputs=-+|
  Viento : Constant  Value=0  OutDataTypeStr=boolean
  Viento_ : Outport
  Ua : Outport  Port=2
  wires:
  Subsistema de modelo de viento/2(W_viento) -> Mux/2
  Altitud/1 -> Subsistema de modelo de viento/1(Altitud)
  Subsistema de modelo de viento/1(V_viento) -> Mux/1, Sum/1
  Viento/1 -> Subsistema de modelo de viento/Enable, Interruptor/2
  Modulo de V_total/1(V_total) -> Subsistema de modelo de viento/2(V_total)
  "U, V, W"/1 -> Sum/2, Modulo de V_total/1("U, V, W")
  "phi, theta, psi"/1 -> R_nb/1
  R_nb/1 -> Subsistema de modelo de viento/3(R_bn)
  Selector/1 -> Ua/1
  Sum/1 -> Selector/1
  Mux/1 -> Producto/2
  Producto/1 -> Viento_/1
  Interruptor/1 -> Producto/1
  Constante/1 -> Interruptor/1
  Constante1/1 -> Interruptor/3

== system Simulador/Motor ==

== system Simulador/Palanca//Teclado ==

== system Simulador/Posicion y actitud ==
  note: Subsistema que calcula la
      | posicion y actitud del UAV.
  "U, V, W" : Inport
  "P, Q, R" : Inport  Port=2
  "phi, theta, psi" : Inport  Port=3
  Al espacio de trabajo : ToWorkspace  VariableName=posicion_NED  SaveFormat=Timeseries  SampleTime=-1
  Demux : Demux  Outputs=3
  Integrador : Integrator  InitialCondition=[0 0 0]
  Integrador1 : Integrator  InitialCondition=[8.12415e-06 0.0301555 270*pi/180]
  Mux1 : Mux  Inputs=2
  Mux2 : Mux  Inputs=3
  Terminador : Terminator
  Velocidades angulares : MATLABFcn  MATLABFcn=velocidades_ang  OutputDimensions=3
  Velocidades lineales : MATLABFcn  MATLABFcn=velocidades_lin  OutputDimensions=3
  "N, E, D" : Outport
  "phi_, theta_, psi_" : Outport  Port=2
  wires:
  Velocidades lineales/1 -> Integrador/1  "V_N, V_E, V_D"
  Velocidades angulares/1 -> Integrador1/1  "W_N, W_E, W_D"
  Mux1/1 -> Velocidades lineales/1  "U, V, W"
  "phi, theta, psi"/1 -> Demux/1, Mux1/2
  Demux/1 -> Mux2/2
  Demux/2 -> Mux2/3
  Mux2/1 -> Velocidades angulares/1  "P, Q, R"
  Demux/3 -> Terminador/1
  Integrador/1 -> "N, E, D"/1, Al espacio de trabajo/1  "N, E, D"
  "P, Q, R"/1 -> Mux2/1
  Integrador1/1 -> "phi_, theta_, psi_"/1  "phi, theta, psi"
  "U, V, W"/1 -> Mux1/1

== system Simulador/Post procesamiento ==
  note: Subsistema que procesa los calculos
      | obtenidos y los prepara para su
      | enrutamiento hacia otros subsistemas.
  Coordenadas geodeticas iniciales : Inport
  "N, E, D" : Inport  Port=2
  "phi, theta, psi" : Inport  Port=3
  Al espacio de trabajo : ToWorkspace  VariableName=posicion_inicial  SaveFormat=Timeseries  SampleTime=-1
  Demux4 : Demux  Outputs=3
  Ganancia : Gain  Gain=-1
  Mux1 : Mux  Inputs=2
  Mux10 : Mux  Inputs=2
  NED a geodeticas : MATLABFcn  MATLABFcn=ned_geodeticas  OutputDimensions=3
  Procesador de actitud : MATLABFcn  MATLABFcn=procesador_actitud  OutputDimensions=3
  Selector : Selector  InputPortWidth=3  Indices=3
  Selector1 : Selector  InputPortWidth=3  Indices=[2 1 3]
  Selector2 : Selector  InputPortWidth=3  Indices=[2 1 3]
  Sum : Sum  Inputs=|++
  Terminador : Terminator
  Terminador1 : Terminator
  Modelo gravitatorio : Outport
  Animacion en Flightgear : Outport  Port=2
  Posicion_NED : Outport  Port=3
  Posion_geodetica_inicial : Outport  Port=4
  Posicion_geodetica : Outport  Port=5
  "phi, theta, psi (procesado)" : Outport  Port=6
  Altitud : Outport  Port=7
  wires:
  Demux4/1 -> Terminador/1
  Demux4/2 -> Terminador1/1
  Demux4/3 -> Ganancia/1
  Ganancia/1 -> Sum/1
  Selector/1 -> Sum/2
  "N, E, D"/1 -> Posicion_NED/1, Mux10/2, Demux4/1
  Coordenadas geodeticas iniciales/1 -> Al espacio de trabajo/1, Posion_geodetica_inicial/1, Selector/1, Mux10/1
  Mux10/1 -> NED a geodeticas/1
  NED a geodeticas/1 -> Selector2/1, Selector1/1, Mux1/1
  Mux1/1 -> Animacion en Flightgear/1
  Selector1/1 -> Posicion_geodetica/1
  Procesador de actitud/1 -> "phi, theta, psi (procesado)"/1, Mux1/2
  "phi, theta, psi"/1 -> Procesador de actitud/1
  Sum/1 -> Altitud/1
  Selector2/1 -> Modelo gravitatorio/1

== system Simulador/Pre visualizacion ==
  note: Subsistema que acondiciona las
      | senales de entrada para su posterior
      | visualizacion en pantalla.
  "U, V, W" : Inport
  "P, Q, R" : Inport  Port=2
  "phi, theta, psi (procesado)" : Inport  Port=3
  "delta_a, delta_e, delta_t" : Inport  Port=4
  Viento : Inport  Port=5
  Altitud : Inport  Port=6
  Densidad : Inport  Port=7
  Al espacio de trabajo1 : ToWorkspace  VariableName=actitud  SaveFormat=Timeseries  SampleTime=-1
  Conversor de angulos{,1..3} (4 alike) : aerolibconvert2/Angle Conversion  IU=rad  OU=deg
  Demux1 : Demux  Outputs=3
  Modulo de Va_total : Subsystem
  Mux : Mux  Inputs=3
  Mux1 : Mux
  Mux2 : Mux
  Mux3 : Mux  Inputs=5
  Selector : Selector  InputPortWidth=6  Indices=[1 2 3]
  Sum : Sum  Inputs=+-|
  Estado : Outport
  Pantalla de estado : Outport  Port=2
  Pantalla de parametros adicionales : Outport  Port=3
  wires:
  Mux1/1 -> Estado/1
  Conversor de angulos2/1 -> Mux/1
  Conversor de angulos3/1 -> Mux/2
  Demux1/2 -> Conversor de angulos3/1
  Demux1/1 -> Conversor de angulos2/1
  Demux1/3 -> Mux/3
  Mux/1 -> Mux2/4
  Mux2/1 -> Pantalla de estado/1
  "delta_a, delta_e, delta_t"/1 -> Demux1/1, Mux1/4
  "phi, theta, psi (procesado)"/1 -> Conversor de angulos1/1, Mux1/3
  "U, V, W"/1 -> Mux1/1, Mux2/1, Sum/1
  Conversor de angulos/1 -> Mux2/2
  "P, Q, R"/1 -> Mux1/2, Conversor de angulos/1
  Viento/1 -> Selector/1
  Sum/1 -> Modulo de Va_total/1("Ua, Va, Wa"), Mux3/1  "Ua, Va, Wa"
  Mux3/1 -> Pantalla de parametros adicionales/1
  Selector/1 -> Mux3/2, Sum/2
  Conversor de angulos1/1 -> Mux2/3, Al espacio de trabajo1/1
  Densidad/1 -> Mux3/5
  Altitud/1 -> Mux3/4
  Modulo de Va_total/1(Va_total) -> Mux3/3

== system Simulador/Rumbo_AP ==

== system Simulador/Velocidad_aerodinamica_AP ==

== system Simulador/Viento ==

== system Simulador/Autopiloto/Activador de controladores ==
  Botones : Inport
  Demux : Demux  Outputs=11
  Interruptor con latch : Subsystem
  Interruptor con latch1 : Subsystem
  Interruptor con latch2 : Subsystem
  Interruptor con latch3 : Subsystem
  Interruptor con latch4 : Subsystem
  Interruptor con latch5 : Subsystem
  Interruptor con latch6 : Subsystem
  Interruptor con latch7 : Subsystem
  Interruptor con latch8 : Subsystem
  Interruptor con latch9 : Subsystem
  Vacio : Outport  PortDimensions=1
  Vacio1 : Outport  Port=2  PortDimensions=1
  Vacio2 : Outport  Port=3  PortDimensions=1
  Vacio3 : Outport  Port=4  PortDimensions=1
  Controlador de phi : Outport  Port=5  PortDimensions=1
  Controlador de psi : Outport  Port=6  PortDimensions=1
  Controlador de theta : Outport  Port=7  PortDimensions=1
  Controlador de h : Outport  Port=8  PortDimensions=1
  Controlador de Uinf mediante theta : Outport  Port=9  PortDimensions=1
  Controlador de Uinf mediante delta_t : Outport  Port=10  PortDimensions=1
  wires:
  Botones/1 -> Demux/1
  Demux/2 -> Interruptor con latch/1(Estado del boton)
  Demux/3 -> Interruptor con latch1/1(Estado del boton)
  Demux/4 -> Interruptor con latch2/1(Estado del boton)
  Demux/5 -> Interruptor con latch3/1(Estado del boton)
  Demux/6 -> Interruptor con latch4/1(Estado del boton)
  Demux/7 -> Interruptor con latch5/1(Estado del boton)
  Demux/8 -> Interruptor con latch6/1(Estado del boton)
  Demux/9 -> Interruptor con latch7/1(Estado del boton)
  Demux/10 -> Interruptor con latch8/1(Estado del boton)
  Demux/11 -> Interruptor con latch9/1(Estado del boton)
  Interruptor con latch9/1(Estado del controlador) -> Controlador de Uinf mediante delta_t/1
  Interruptor con latch8/1(Estado del controlador) -> Controlador de Uinf mediante theta/1
  Interruptor con latch6/1(Estado del controlador) -> Controlador de theta/1
  Interruptor con latch4/1(Estado del controlador) -> Controlador de phi/1
  Interruptor con latch/1(Estado del controlador) -> Vacio/1
  Interruptor con latch1/1(Estado del controlador) -> Vacio1/1
  Interruptor con latch2/1(Estado del controlador) -> Vacio2/1
  Interruptor con latch3/1(Estado del controlador) -> Vacio3/1
  Demux/1 -> Interruptor con latch/2(Reinicio), Interruptor con latch1/2(Reinicio), Interruptor con latch2/2(Reinicio), Interruptor con latch3/2(Reinicio), Interruptor con latch4/2(Reinicio), Interruptor con latch5/2(Reinicio), Interruptor con latch6/2(Reinicio), Interruptor con latch7/2(Reinicio), Interruptor con latch9/2(Reinicio), Interruptor con latch8/2(Reinicio)
  Interruptor con latch5/1(Estado del controlador) -> Controlador de psi/1
  Interruptor con latch7/1(Estado del controlador) -> Controlador de h/1

== system Simulador/Autopiloto/Calculador de coeficientes aerodinamicos (alpha) ==
  Viento : Inport
  "U, V, W" : Inport  Port=2
  Modelo aerodinamico : Inport  Port=3
  Constante : Constant  Value=0
  Constante1 : Constant  Value=1e-16
  Constante2 : Constant  Value=[0 0 0 0 0]
  Division : Product  Inputs=*/
  Funcion trigonometrica : Trigonometry  Operator=atan
  Modelo aerodinamico del X8 : MATLABFcn  MATLABFcn=x8_aero  OutputDimensions=6
  Modulo de Va_total : Subsystem
  Mux : Mux  Inputs=6
  Selector : Selector  InputPortWidth=6  Indices=[1 2 3]
  Selector2 : Selector  InputPortWidth=3  Indices=3
  Selector3 : Selector  InputPortWidth=3
  Sigma : MATLABFcn  MATLABFcn=sigmoid  OutputDimensions=1
  Sum : Sum  Inputs=|-+
  Sum3 : Sum  Inputs=|++
  Coeficientes aerodinamicos (alpha) : Outport
  wires:
  Viento/1 -> Selector/1
  "U, V, W"/1 -> Sum/2
  Selector/1 -> Sum/1  "Uv, Vv, Wv"
  Sum/1 -> Selector3/1, Selector2/1, Modulo de Va_total/1("Ua, Va, Wa")  "Ua, Va, Wa"
  Selector2/1 -> Division/1
  Sum3/1 -> Division/2
  Division/1 -> Funcion trigonometrica/1
  Modulo de Va_total/1(Va_total) -> Mux/3  "Uinf"
  Funcion trigonometrica/1 -> Sigma/1, Mux/1  "alpha"
  Mux/1 -> Modelo aerodinamico del X8/1
  Modelo aerodinamico del X8/1 -> Coeficientes aerodinamicos (alpha)/1
  Constante1/1 -> Sum3/2
  Selector3/1 -> Sum3/1
  Constante/1 -> Mux/2
  Modelo aerodinamico/1 -> Mux/6
  Sigma/1 -> Mux/5  "sigma"
  Constante2/1 -> Mux/4

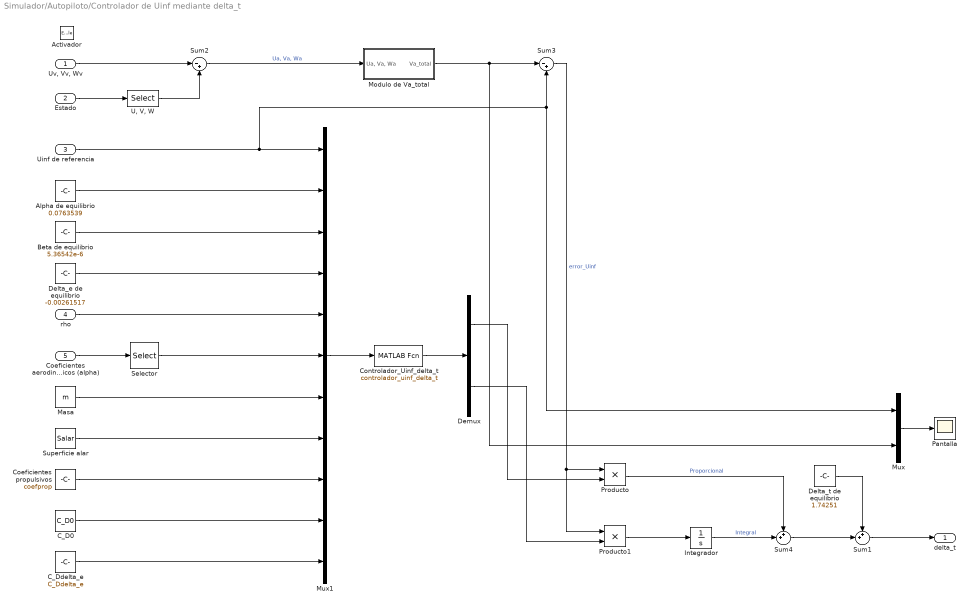
== system Simulador/Autopiloto/Controlador de Uinf mediante delta_t ==
  "Uv, Vv, Wv" : Inport
  "Estado " : Inport  Port=2
  Uinf de referencia : Inport  Port=3
  rho : Inport  Port=4
  Coeficientes aerodinamicos (alpha) : Inport  Port=5
  Activador : EnablePort
  Alpha de equilibrio : Constant  Value=0.0763539
  Beta de equilibrio : Constant  Value=5.36542e-6
  C_D0 : Constant  Value=C_D0
  C_Ddelta_e : Constant  Value=C_Ddelta_e
  Coeficientes propulsivos : Constant  Value=coefprop
  Controlador_Uinf_delta_t : MATLABFcn  MATLABFcn=controlador_uinf_delta_t  OutputDimensions=2
  Delta_e de equilibrio : Constant  Value=-0.00261517
  Delta_t de equilibrio : Constant  Value=1.74251
  Demux : Demux  Outputs=2
  Integrador : Integrator
  Masa : Constant  Value=m
  Modulo de Va_total : Subsystem
  Mux : Mux  Inputs=2
  Mux1 : Mux  Inputs=11
  Pantalla : Scope
      settings: TimeRange=9.663330776874403  YMin=25  YMax=25.0011  SaveName=ScopeData2
  Producto : Product
  Producto1 : Product
  Selector : Selector  InputPortWidth=6  Indices=2
  Sum1 : Sum  Inputs=++|
  Sum2 : Sum  Inputs=|-+
  Sum3 : Sum  Inputs=|-+
  Sum4 : Sum  Inputs=++|
  Superficie alar : Constant  Value=Salar
  "U, V, W" : Selector  InputPortWidth=12  Indices=[1 2 3]
      settings: AttributesFormatString=(Joystick - dependent)
  delta_t : Outport
  wires:
  Controlador_Uinf_delta_t/1 -> Demux/1
  Producto/1 -> Sum4/1  "Proporcional"
  Demux/1 -> Producto/2
  Demux/2 -> Producto1/2
  Mux/1 -> Pantalla/1
  Mux1/1 -> Controlador_Uinf_delta_t/1
  Integrador/1 -> Sum4/2  "Integral"
  Producto1/1 -> Integrador/1
  Sum1/1 -> delta_t/1
  Delta_t de equilibrio/1 -> Sum1/1
  Sum4/1 -> Sum1/2
  "U, V, W"/1 -> Sum2/2
  "Uv, Vv, Wv"/1 -> Sum2/1
  Sum2/1 -> Modulo de Va_total/1("Ua, Va, Wa")  "Ua, Va, Wa"
  "Estado "/1 -> "U, V, W"/1
  Modulo de Va_total/1(Va_total) -> Sum3/1, Mux/2
  Sum3/1 -> Producto1/1, Producto/1  "error_Uinf"
  Uinf de referencia/1 -> Sum3/2, Mux/1, Mux1/1
  Alpha de equilibrio/1 -> Mux1/2
  Beta de equilibrio/1 -> Mux1/3
  Delta_e de equilibrio/1 -> Mux1/4
  rho/1 -> Mux1/5
  Coeficientes aerodinamicos (alpha)/1 -> Selector/1
  Selector/1 -> Mux1/6
  C_D0/1 -> Mux1/10
  C_Ddelta_e/1 -> Mux1/11
  Masa/1 -> Mux1/7
  Superficie alar/1 -> Mux1/8
  Coeficientes propulsivos/1 -> Mux1/9

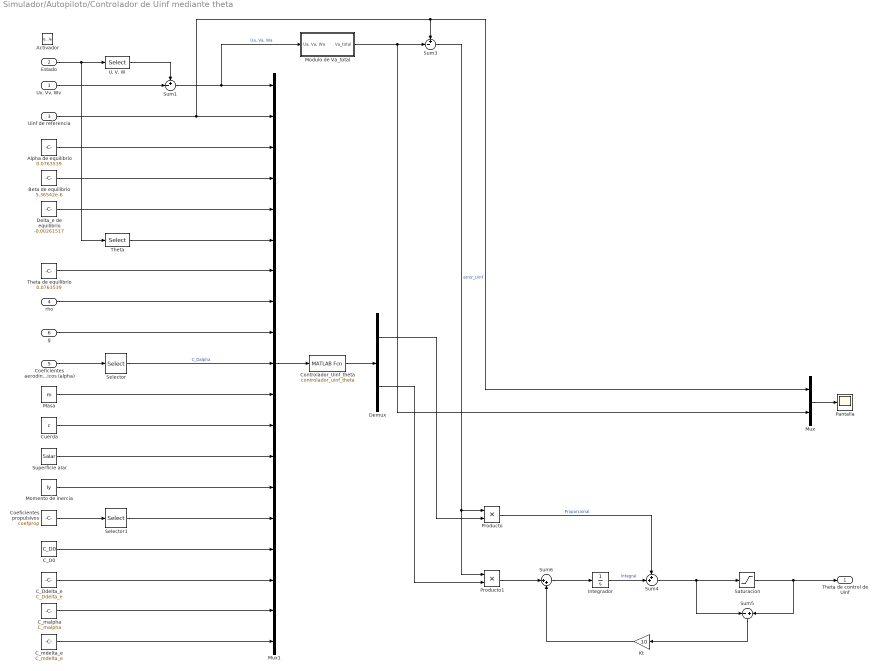
== system Simulador/Autopiloto/Controlador de Uinf mediante theta ==
  "Uv, Vv, Wv" : Inport
  "Estado " : Inport  Port=2
  Uinf de referencia : Inport  Port=3
  rho : Inport  Port=4
  Coeficientes aerodinamicos (alpha) : Inport  Port=5
  g : Inport  Port=6
  Activador : EnablePort
  Alpha de equilibrio : Constant  Value=0.0763539
  Beta de equilibrio : Constant  Value=5.36542e-6
  C_D0 : Constant  Value=C_D0
  C_Ddelta_e : Constant  Value=C_Ddelta_e
  C_malpha : Constant  Value=C_malpha
  C_mdelta_e : Constant  Value=C_mdelta_e
  Coeficientes propulsivos : Constant  Value=coefprop
  Controlador_Uinf_theta : MATLABFcn  MATLABFcn=controlador_uinf_theta  OutputDimensions=2
  Cuerda : Constant  Value=c
  Delta_e de equilibrio : Constant  Value=-0.00261517
  Demux : Demux  Outputs=2
  Integrador : Integrator
  Kt : Gain  Gain=10
  Masa : Constant  Value=m
  Modulo de Va_total : Subsystem
  Momento de inercia : Constant  Value=Iy
  Mux : Mux  Inputs=2
  Mux1 : Mux  Inputs=19
  Pantalla : Scope
      settings: TimeRange=9.663330776874403  YMin=14.5  YMax=15.9  SaveName=ScopeData2
  Producto : Product
  Producto1 : Product
  Saturacion : Saturate  UpperLimit=30*pi/180  LowerLimit=0
  Selector : Selector  InputPortWidth=6  Indices=2
  Selector1 : Selector  InputPortWidth=2  Indices=2
  Sum1 : Sum  Inputs=+-|
  Sum3 : Sum  Inputs=+-|
  Sum4 : Sum  Inputs=++|
  Sum5 : Sum  Inputs=-|+
  Sum6 : Sum  Inputs=|++
  Superficie alar : Constant  Value=Salar
  Theta : Selector  InputPortWidth=12  Indices=8
      settings: AttributesFormatString=(Joystick - dependent)
  Theta de equilibrio : Constant  Value=0.0763539
  "U, V, W" : Selector  InputPortWidth=12  Indices=[1 2 3]
      settings: AttributesFormatString=(Joystick - dependent)
  Theta de control de Uinf : Outport
  wires:
  Controlador_Uinf_theta/1 -> Demux/1
  Producto/1 -> Sum4/1  "Proporcional"
  Producto1/1 -> Sum6/1
  Demux/1 -> Producto/2
  Demux/2 -> Producto1/2
  Mux/1 -> Pantalla/1
  Mux1/1 -> Controlador_Uinf_theta/1
  Uinf de referencia/1 -> Mux/1, Sum3/1, Mux1/2
  Alpha de equilibrio/1 -> Mux1/3
  Saturacion/1 -> Sum5/2, Theta de control de Uinf/1
  Integrador/1 -> Sum4/2  "Integral"
  Sum5/1 -> Kt/1
  Sum6/1 -> Integrador/1
  Sum4/1 -> Saturacion/1, Sum5/1
  Kt/1 -> Sum6/2
  Theta/1 -> Mux1/6
  Theta de equilibrio/1 -> Mux1/7
  Delta_e de equilibrio/1 -> Mux1/5
  Beta de equilibrio/1 -> Mux1/4
  "Estado "/1 -> "U, V, W"/1, Theta/1
  Sum1/1 -> Modulo de Va_total/1("Ua, Va, Wa"), Mux1/1  "Ua, Va, Wa"
  rho/1 -> Mux1/8
  Sum3/1 -> Producto1/1, Producto/1  "error_Uinf"
  Modulo de Va_total/1(Va_total) -> Sum3/2, Mux/2
  "Uv, Vv, Wv"/1 -> Sum1/2
  "U, V, W"/1 -> Sum1/1
  Coeficientes aerodinamicos (alpha)/1 -> Selector/1
  Selector/1 -> Mux1/10  "C_Dalpha"
  Masa/1 -> Mux1/11
  Cuerda/1 -> Mux1/12
  Superficie alar/1 -> Mux1/13
  C_D0/1 -> Mux1/16
  C_Ddelta_e/1 -> Mux1/17
  C_malpha/1 -> Mux1/18
  C_mdelta_e/1 -> Mux1/19
  Coeficientes propulsivos/1 -> Selector1/1
  Selector1/1 -> Mux1/15
  Momento de inercia/1 -> Mux1/14
  g/1 -> Mux1/9

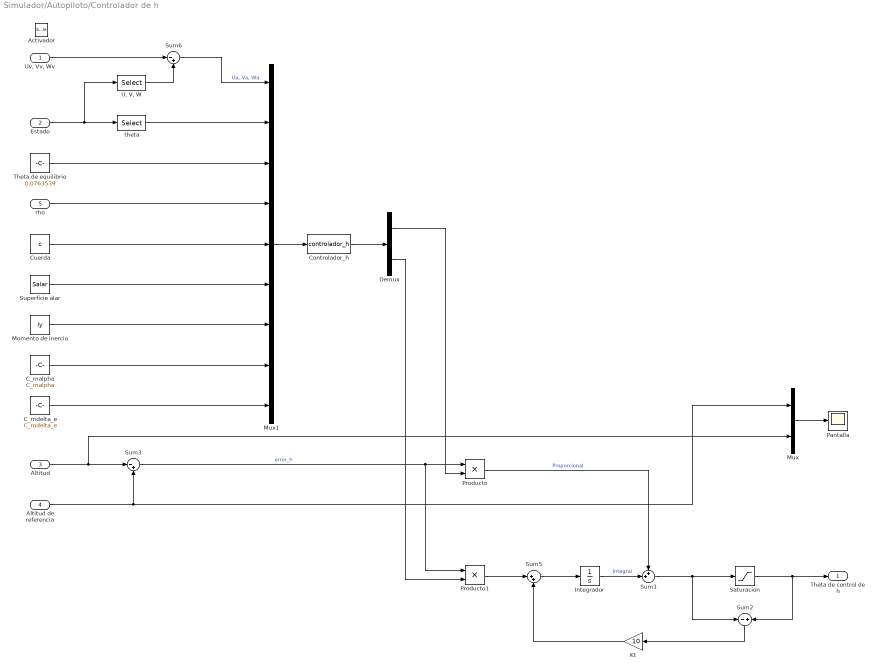
== system Simulador/Autopiloto/Controlador de h ==
  "Uv, Vv, Wv" : Inport
  "Estado " : Inport  Port=2
  Altitud : Inport  Port=3
  Altitud de referencia : Inport  Port=4
  rho : Inport  Port=5
  Activador : EnablePort
  C_malpha : Constant  Value=C_malpha
  C_mdelta_e : Constant  Value=C_mdelta_e
  Controlador_h : MATLABFcn  MATLABFcn=controlador_h  OutputDimensions=2
  Cuerda : Constant  Value=c
  Demux : Demux  Outputs=2
  Integrador : Integrator
  Kt : Gain  Gain=10
  Momento de inercia : Constant  Value=Iy
  Mux : Mux  Inputs=2
  Mux1 : Mux  Inputs=9
  Pantalla : Scope
      settings: TimeRange=9.663330776874403  YMin=154  YMax=160  SaveName=ScopeData3
  Producto : Product
  Producto1 : Product
  Saturacion : Saturate  UpperLimit=30*pi/180  LowerLimit=-5*pi/180
  Sum1 : Sum  Inputs=++|
  Sum2 : Sum  Inputs=-|+
  Sum3 : Sum  Inputs=|-+
  Sum5 : Sum  Inputs=|++
  Sum6 : Sum  Inputs=|-+
  Superficie alar : Constant  Value=Salar
  Theta de equilibrio : Constant  Value=0.0763539
  "U, V, W" : Selector  InputPortWidth=12  Indices=[1 2 3]
      settings: AttributesFormatString=(Joystick - dependent)
  theta : Selector  InputPortWidth=12  Indices=8
      settings: AttributesFormatString=(Joystick - dependent)
  Theta de control de h : Outport
  wires:
  "Estado "/1 -> theta/1, "U, V, W"/1
  Controlador_h/1 -> Demux/1
  Producto/1 -> Sum1/1  "Proporcional"
  Integrador/1 -> Sum1/2  "Integral"
  Kt/1 -> Sum5/2
  Sum2/1 -> Kt/1
  Demux/2 -> Producto1/2
  Demux/1 -> Producto/2
  Producto1/1 -> Sum5/1
  Sum5/1 -> Integrador/1
  Mux1/1 -> Controlador_h/1
  Saturacion/1 -> Theta de control de h/1, Sum2/2
  Theta de equilibrio/1 -> Mux1/3
  theta/1 -> Mux1/2
  Altitud/1 -> Mux/2, Sum3/1
  Sum3/1 -> Producto/1, Producto1/1  "error_h"
  Altitud de referencia/1 -> Sum3/2, Mux/1
  Sum1/1 -> Saturacion/1, Sum2/1
  "U, V, W"/1 -> Sum6/2
  "Uv, Vv, Wv"/1 -> Sum6/1
  Sum6/1 -> Mux1/1  "Ua, Va, Wa"
  Mux/1 -> Pantalla/1
  rho/1 -> Mux1/4
  Cuerda/1 -> Mux1/5
  Superficie alar/1 -> Mux1/6
  Momento de inercia/1 -> Mux1/7
  C_malpha/1 -> Mux1/8
  C_mdelta_e/1 -> Mux1/9
